simulink model "state_flow"  (R2020a)
settings: Solver=VariableStepAuto  StartTime=0.0  StopTime=10.0  RelTol=1e-3
settings Model: Creator=naina  LastModifiedBy=naina

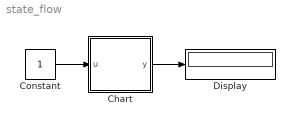
== system state_flow ==
  Chart : Stateflow chart  TreatAsAtomicUnit=on
  Constant : Constant
  Display : Display
  wires:
  Constant/1 -> Chart/1(u)
  Chart/1(y) -> Display/1

== stateflow chart state_flow/Chart ==
  state ON
    entry: y =-3;
  state OFF
    entry: y = 3;
  (default) -> ON
  ON -> OFF : [u>=1]
  OFF -> ON : [u<1]
  data: u input; y output
